simulink model "plant"  (R2023b)
settings: Solver=FixedStepAuto  StartTime=0.0  StopTime=SIMTIME  FixedStep=SIMSTEP  RelTol=1e-3
values from neighbouring files (symbols this model uses):
  A = [z33,    eye(3) ... (first row only)    [plant.m]
  B = [z33, inv(M)]'    [plant.m]
  beta_c = deg2rad(1)    [plant.m]
  bias = [1e5;0;0]    [plant.m]
  bias_switch = -1    [plant.m]
  Bv = [z33 z33 ... (first row only)    [plant.m]
  C = [eye(3,6)]    [plant.m]
  ref = zeros(3,1)    [plant.m]
  V_curr = 2    [plant.m]
  V_wind = 0    [plant.m]
  wave_ampl = [0, 0, 0]    [plant.m]
  wave_length = [70 70 70]    [plant.m]
  x0 = zeros(n_states, 1)    [plant.m]
undefined symbols (not defined in the file or in its folder): ocean_coeff, wind_coeff
settings Model: Creator=X20  LastModifiedBy=Lorenzo-Desk
settings DataIOCC: ReturnWorkspaceOutputs=off

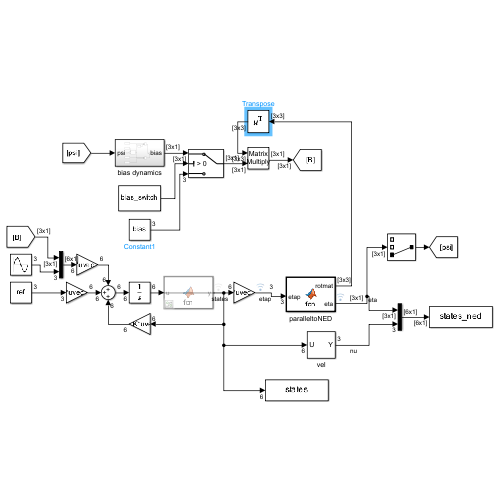
[thumbnail: Simulink's stored preview of the top-level diagram]
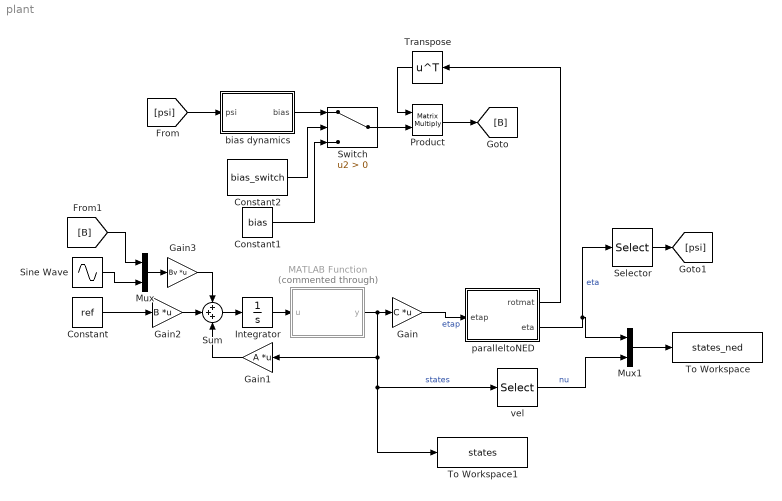
== system plant ==
  Constant : Constant  Value=ref
  Constant1 : Constant  Value=bias
  Constant2 : Constant  Value=bias_switch
  Gain : Gain  Gain=C  Multiplication=Matrix(K*u) (u vector)
  Gain1 : Gain  Gain=A  Multiplication=Matrix(K*u) (u vector)
  Gain2 : Gain  Gain=B  Multiplication=Matrix(K*u) (u vector)
  Gain3 : Gain  Gain=Bv  Multiplication=Matrix(K*u) (u vector)
  Integrator : Integrator  InitialCondition=x0
  MATLAB Function : MATLAB Function  Commented=through  TreatAsAtomicUnit=on
  Mux : Mux  Inputs=2
  Mux1 : Mux  Inputs=2
  Product : Product  Multiplication=Matrix(*)
  Selector : Selector  InputPortWidth=3  IndexOptions=Index vector (dialog)  Indices=[3]  OutputSizes=1
  Sine Wave : Sin  Amplitude=wave_ampl  Frequency=1./wave_length  SampleTime=0
  Sum : Sum  Inputs=+++
  Switch : Switch  Criteria=u2 > Threshold  SaturateOnIntegerOverflow=off  InputSameDT=off
  To Workspace : ToWorkspace  VariableName=states_ned  SaveFormat=Timeseries  SampleTime=-1
  To Workspace1 : ToWorkspace  VariableName=states  SaveFormat=Timeseries  SampleTime=-1
  Transpose : Math  Operator=transpose
  bias dynamics : Subsystem
  paralleltoNED : MATLAB Function  TreatAsAtomicUnit=on
  vel : Selector  InputPortWidth=6  IndexOptions=Index vector (dialog)  Indices=[4 5 6]  OutputSizes=1
  wires:
  Sum/1 -> Integrator/1
  Gain1/1 -> Sum/3
  Constant/1 -> Gain2/1
  Integrator/1 -> MATLAB Function/1(u)
  Gain2/1 -> Sum/2
  Mux/1 -> Gain3/1
  Gain3/1 -> Sum/1
  [B] -> Mux/1
  Sine Wave/1 -> Mux/2
  [psi] -> bias dynamics/1(psi)
  Gain/1 -> paralleltoNED/1(etap)  "etap"
  Mux1/1 -> To Workspace/1
  paralleltoNED/2(eta) -> Selector/1, Mux1/1  "eta"
  vel/1 -> Mux1/2  "nu"
  Selector/1 -> [psi]
  paralleltoNED/1(rotmat) -> Transpose/1
  Transpose/1 -> Product/1
  MATLAB Function/1(y) -> Gain/1, To Workspace1/1, vel/1, Gain1/1  "states"
  Constant1/1 -> Switch/3
  Constant2/1 -> Switch/2
  Product/1 -> [B]
  Switch/1 -> Product/2
  bias dynamics/1(bias) -> Switch/1

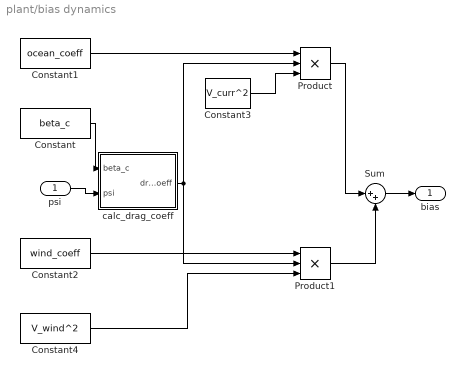
== system plant/bias dynamics ==
  psi : Inport
  Constant : Constant  Value=beta_c
  Constant1 : Constant  Value=ocean_coeff
  Constant2 : Constant  Value=wind_coeff
  Constant3 : Constant  Value=V_curr^2
  Constant4 : Constant  Value=V_wind^2
  Product : Product  Inputs=3
  Product1 : Product  Inputs=3
  Sum : Sum  Inputs=|++
  calc_drag_coeff : MATLAB Function  TreatAsAtomicUnit=on
  bias : Outport
  wires:
  psi/1 -> calc_drag_coeff/2(psi)
  Constant/1 -> calc_drag_coeff/1(beta_c)
  Constant4/1 -> Product1/3
  Product/1 -> Sum/1
  Product1/1 -> Sum/2
  Sum/1 -> bias/1
  Constant1/1 -> Product/1
  calc_drag_coeff/1(drag_coeff) -> Product1/2, Product/2
  Constant3/1 -> Product/3
  Constant2/1 -> Product1/1

== matlab function plant/paralleltoNED ==
  data: rotmat output; etap input; eta output
function [rotmat, eta] = fcn(etap)
    psip = etap(3);
    rotmat = [cos(psip), -sin(psip), 0; 
              sin(psip),  cos(psip), 0;
                      0,          0, 1];
    eta = rotmat*etap;
end

== matlab function plant/MATLAB Function ==
  data: u input; y output
function y = fcn(u)
    u(3) = wrapTo2Pi(u(3)) - pi;
    y = u;
end

== matlab function plant/bias dynamics/calc_drag_coeff ==
  data: beta_c input; drag_coeff output; psi input
function drag_coeff = fcn(beta_c, psi)
    angle_of_attack = psi-beta_c-pi;
    cx = 0.7;
    cy = 0.8; 
    cn = 0.15;
    Cx = -cx*cos(angle_of_attack);
    Cy = cy*sin(angle_of_attack);
    Cn = cn*sin(2*angle_of_attack);
    drag_coeff = [Cx, Cy, Cn]';
end
